simulink model "CubeX_LQR_2D_READ"  (R2016b)
settings: Solver=VariableStepAuto  StartTime=0.0  StopTime=inf  RelTol=1e-3
settings Model: Creator=Wall  LastModifiedBy=Wall

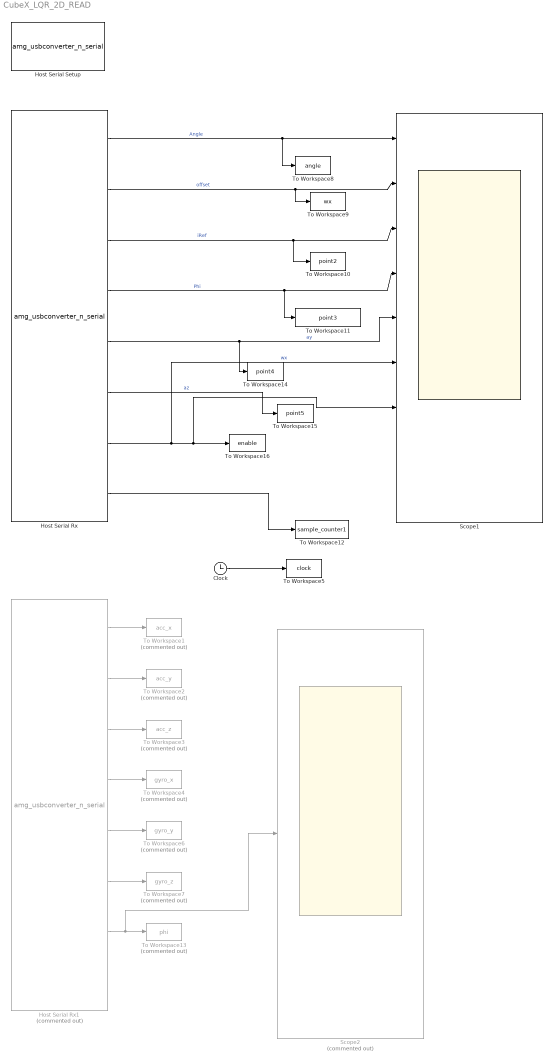
== system CubeX_LQR_2D_READ ==
  Clock : Clock
  Host Serial Rx : S-Function  Priority=1  FunctionName=amg_usbconverter_n_serial  Parameters=configuration,port,transfer,baudrate,stopbit,inputtype,outputtype,binheaderarray,binterminatorarray,asciiheader,asciiterminator,bindatalength,packetmode,timeout,sampletime,initialvalues,blockid  SFunctionDeploymentMode=off  EnableBusSupport=off  mask(amg_usbconverter_n_serial){configuration=Rx, port=COM3, baudrate=115200, databits=8, parity=None, stopbit=1, flowcontrol=None, advanceoptions=off, rxbuffersize=2048, txbuffersize=2048, transfer=Blocking, enableinitial=off, initialvalues=[], timeout=5, packetmode=Binary, binheader='0E 0E', binterminator='0A 0A', porttype_double=8, porttype_single=0, porttype_int8=0, porttype_uint8=0, porttype_int16=0, porttype_uint16=0, porttype_int32=0, porttype_uint32=0, asciiformat='%d,%f', rx_asciiterminator=LF (0x0A - "\n"), tx_asciiterminator=LF (0x0A - "\n"), inputtype=[0], outputtype=[8  0 0 0 0 0 0 0 0], binheaderarray=[2 14  14], binterminatorarray=[2 10  10], bindatalength=64, asciiheader=['%d,%f' uint8(10)], asciiterminator=[1 10], sampletime=0.002, sampletimestr=, blockid=HostSerialRx}
      mask prompts: baudrate "Baud rate (bps)"; databits "Data bits"; stopbit "Stop bit"; flowcontrol "Hardware flow control"; advanceoptions "Advance options"; rxbuffersize "Rx buffer size (bytes)"; txbuffersize "Tx buffer size (bytes)"; enableinitial "Enable initial value  (Closed loop HIL test)"; initialvalues "Initial values"; timeout "Wait time-out (Seconds)"; packetmode "Packet mode"; binheader "Binary header (example: '7E 7E')"; binterminator "Binary terminator (example: '03 03')"; porttype_double "Number of data port, type DOUBLE"; porttype_single "Number of data port, type SINGLE"; porttype_int8 "Number of data port, type INT8"; porttype_uint8 "Number of data port, type UINT8"; porttype_int16 "Number of data port, type INT16"; porttype_uint16 "Number of data port, type UINT16"; porttype_int32 "Number of data port, type INT32"; porttype_uint32 "Number of data port, type UINT32"; asciiformat "Ascii format"; rx_asciiterminator "End of packet"; tx_asciiterminator "End of packet"; inputtype "Input data type"; outputtype "Output data type"; binheaderarray "Binary header"; binterminatorarray "Binary terminator"; bindatalength "Binary data length"; asciiheader "Ascii header (printf format)"; asciiterminator "Ascii terminator"; sampletime "Sample time (sec)"; sampletimestr "Compiled sample time (sec) in string"
      mask help:
      | Enable initial value (Closed loop HIL test):
      |  - Checked: The block will return a initial value (constant) at first time step.
      |  - Unchecked: Normal operation, the block waiting for matched packet data before return value.
      mask init:
      | amg_usbconverter_n_serial_callback('init');
      mask Help: web(fullfile(waijungdocroot,'amg_usbconverter_n_uart.htm'), '-browser')
      mask TypeOptions configuration: Setup | Tx | Rx
      mask Callback configuration: amg_usbconverter_n_serial_callback('configuration');
      mask TypeOptions port: COM3
      mask Callback port: amg_usbconverter_n_serial_callback('port');
      mask Callback baudrate: amg_usbconverter_n_serial_callback('baudrate');
      mask TypeOptions databits: 8
      mask TypeOptions parity: None
      mask TypeOptions stopbit: 1 | 1.5 | 2
      mask TypeOptions flowcontrol: None | RTS | CTS | RTS/CTS
      mask Callback flowcontrol: amg_usbconverter_n_serial_callback('flowcontrol');
      mask Callback advanceoptions: amg_usbconverter_n_serial_callback('advanceoptions');
      mask TypeOptions rxbuffersize: 16 | 32 | 64 | 128 | 256 | 512 | 1024 | 2048
      mask TypeOptions txbuffersize: 16 | 32 | 64 | 128 | 256 | 512 | 1024 | 2048
      mask TypeOptions transfer: Blocking | Non-Blocking
      mask Callback transfer: amg_usbconverter_n_serial_callback('transfer');
      mask Callback enableinitial: amg_usbconverter_n_serial_callback('enableinitial');
      mask Callback initialvalues: amg_usbconverter_n_serial_callback('initialvalues');
      mask TypeOptions packetmode: Ascii | Binary
      mask Callback packetmode: amg_usbconverter_n_serial_callback('packetmode');
      mask Callback binheader: amg_usbconverter_n_serial_callback('binheader');
      mask Callback binterminator: amg_usbconverter_n_serial_callback('binterminator');
      mask Callback porttype_double: amg_usbconverter_n_serial_callback('porttype');
      mask Callback porttype_single: amg_usbconverter_n_serial_callback('porttype');
      mask Callback porttype_int8: amg_usbconverter_n_serial_callback('porttype');
      mask Callback porttype_uint8: amg_usbconverter_n_serial_callback('porttype');
      mask Callback porttype_int16: amg_usbconverter_n_serial_callback('porttype');
      mask Callback porttype_uint16: amg_usbconverter_n_serial_callback('porttype');
      mask Callback porttype_int32: amg_usbconverter_n_serial_callback('porttype');
      mask Callback porttype_uint32: amg_usbconverter_n_serial_callback('porttype');
      mask Callback asciiformat: amg_usbconverter_n_serial_callback('asciiformat');
      mask TypeOptions rx_asciiterminator: CR (0x0D - "\r") | LF (0x0A - "\n") | CRLF (0x0D 0x0A - "\r\n")
      mask Callback rx_asciiterminator: amg_usbconverter_n_serial_callback('rx_asciiterminator');
      mask TypeOptions tx_asciiterminator: CR (0x0D - "\r") | LF (0x0A - "\n") | CRLF (0x0D 0x0A - "\r\n") | None
      mask Callback tx_asciiterminator: amg_usbconverter_n_serial_callback('tx_asciiterminator');
      mask Callback sampletime: amg_usbconverter_n_serial_callback('sampletime');
      mask Callback sampletimestr: amg_usbconverter_n_serial_callback('sampletimestr');
      mask Callback blockid: amg_usbconverter_n_serial_callback('blockid');
      mask Display: text(0.05, 0.5, 'Port: COM3\nPacket: Binary\nTransfer: Blocking\nTs (sec): 0.002','ver','middle','hor','left');port_label('output', 1,'double');port_label('output', 2,'double');port_label('output', 3,'double');port_label('output', 4,'double');port_label('output', 5,'double');port_label('output', 6,'double');port_label('output', 7,'double');port_label('output', 8,'double');
  Host Serial Rx1 : S-Function  Priority=1  Commented=on  FunctionName=amg_usbconverter_n_serial  Parameters=configuration,port,transfer,baudrate,stopbit,inputtype,outputtype,binheaderarray,binterminatorarray,asciiheader,asciiterminator,bindatalength,packetmode,timeout,sampletime,initialvalues,blockid  SFunctionDeploymentMode=off  EnableBusSupport=off  mask(amg_usbconverter_n_serial){configuration=Rx, port=COM3, baudrate=115200, databits=8, parity=None, stopbit=1, flowcontrol=None, advanceoptions=off, rxbuffersize=2048, txbuffersize=2048, transfer=Blocking, enableinitial=off, initialvalues=[], timeout=5, packetmode=Binary, binheader='0E 0E', binterminator='0A 0A', porttype_double=8, porttype_single=0, porttype_int8=0, porttype_uint8=0, porttype_int16=0, porttype_uint16=0, porttype_int32=0, porttype_uint32=0, asciiformat='%d,%f', rx_asciiterminator=LF (0x0A - "\n"), tx_asciiterminator=LF (0x0A - "\n"), inputtype=[0], outputtype=[8  0 0 0 0 0 0 0 0], binheaderarray=[2 14  14], binterminatorarray=[2 10  10], bindatalength=64, asciiheader=['%d,%f' uint8(10)], asciiterminator=[1 10], sampletime=0.002, sampletimestr=, blockid=HostSerialRx1}
      mask prompts: baudrate "Baud rate (bps)"; databits "Data bits"; stopbit "Stop bit"; flowcontrol "Hardware flow control"; advanceoptions "Advance options"; rxbuffersize "Rx buffer size (bytes)"; txbuffersize "Tx buffer size (bytes)"; enableinitial "Enable initial value  (Closed loop HIL test)"; initialvalues "Initial values"; timeout "Wait time-out (Seconds)"; packetmode "Packet mode"; binheader "Binary header (example: '7E 7E')"; binterminator "Binary terminator (example: '03 03')"; porttype_double "Number of data port, type DOUBLE"; porttype_single "Number of data port, type SINGLE"; porttype_int8 "Number of data port, type INT8"; porttype_uint8 "Number of data port, type UINT8"; porttype_int16 "Number of data port, type INT16"; porttype_uint16 "Number of data port, type UINT16"; porttype_int32 "Number of data port, type INT32"; porttype_uint32 "Number of data port, type UINT32"; asciiformat "Ascii format"; rx_asciiterminator "End of packet"; tx_asciiterminator "End of packet"; inputtype "Input data type"; outputtype "Output data type"; binheaderarray "Binary header"; binterminatorarray "Binary terminator"; bindatalength "Binary data length"; asciiheader "Ascii header (printf format)"; asciiterminator "Ascii terminator"; sampletime "Sample time (sec)"; sampletimestr "Compiled sample time (sec) in string"
      mask help:
      | Enable initial value (Closed loop HIL test):
      |  - Checked: The block will return a initial value (constant) at first time step.
      |  - Unchecked: Normal operation, the block waiting for matched packet data before return value.
      mask init:
      | amg_usbconverter_n_serial_callback('init');
      mask Help: web(fullfile(waijungdocroot,'amg_usbconverter_n_uart.htm'), '-browser')
      mask TypeOptions configuration: Setup | Tx | Rx
      mask Callback configuration: amg_usbconverter_n_serial_callback('configuration');
      mask TypeOptions port: COM3
      mask Callback port: amg_usbconverter_n_serial_callback('port');
      mask Callback baudrate: amg_usbconverter_n_serial_callback('baudrate');
      mask TypeOptions databits: 8
      mask TypeOptions parity: None
      mask TypeOptions stopbit: 1 | 1.5 | 2
      mask TypeOptions flowcontrol: None | RTS | CTS | RTS/CTS
      mask Callback flowcontrol: amg_usbconverter_n_serial_callback('flowcontrol');
      mask Callback advanceoptions: amg_usbconverter_n_serial_callback('advanceoptions');
      mask TypeOptions rxbuffersize: 16 | 32 | 64 | 128 | 256 | 512 | 1024 | 2048
      mask TypeOptions txbuffersize: 16 | 32 | 64 | 128 | 256 | 512 | 1024 | 2048
      mask TypeOptions transfer: Blocking | Non-Blocking
      mask Callback transfer: amg_usbconverter_n_serial_callback('transfer');
      mask Callback enableinitial: amg_usbconverter_n_serial_callback('enableinitial');
      mask Callback initialvalues: amg_usbconverter_n_serial_callback('initialvalues');
      mask TypeOptions packetmode: Ascii | Binary
      mask Callback packetmode: amg_usbconverter_n_serial_callback('packetmode');
      mask Callback binheader: amg_usbconverter_n_serial_callback('binheader');
      mask Callback binterminator: amg_usbconverter_n_serial_callback('binterminator');
      mask Callback porttype_double: amg_usbconverter_n_serial_callback('porttype');
      mask Callback porttype_single: amg_usbconverter_n_serial_callback('porttype');
      mask Callback porttype_int8: amg_usbconverter_n_serial_callback('porttype');
      mask Callback porttype_uint8: amg_usbconverter_n_serial_callback('porttype');
      mask Callback porttype_int16: amg_usbconverter_n_serial_callback('porttype');
      mask Callback porttype_uint16: amg_usbconverter_n_serial_callback('porttype');
      mask Callback porttype_int32: amg_usbconverter_n_serial_callback('porttype');
      mask Callback porttype_uint32: amg_usbconverter_n_serial_callback('porttype');
      mask Callback asciiformat: amg_usbconverter_n_serial_callback('asciiformat');
      mask TypeOptions rx_asciiterminator: CR (0x0D - "\r") | LF (0x0A - "\n") | CRLF (0x0D 0x0A - "\r\n")
      mask Callback rx_asciiterminator: amg_usbconverter_n_serial_callback('rx_asciiterminator');
      mask TypeOptions tx_asciiterminator: CR (0x0D - "\r") | LF (0x0A - "\n") | CRLF (0x0D 0x0A - "\r\n") | None
      mask Callback tx_asciiterminator: amg_usbconverter_n_serial_callback('tx_asciiterminator');
      mask Callback sampletime: amg_usbconverter_n_serial_callback('sampletime');
      mask Callback sampletimestr: amg_usbconverter_n_serial_callback('sampletimestr');
      mask Callback blockid: amg_usbconverter_n_serial_callback('blockid');
      mask Display: text(0.05, 0.5, 'Port: COM3\nPacket: Binary\nTransfer: Blocking\nTs (sec): -1','ver','middle','hor','left');port_label('output', 1,'double');port_label('output', 2,'double');port_label('output', 3,'double');port_label('output', 4,'double');port_label('output', 5,'double');port_label('output', 6,'double');port_label('output', 7,'double');port_label('output', 8,'double');
  Host Serial Setup : S-Function  Priority=1  FunctionName=amg_usbconverter_n_serial  Parameters=configuration,port,transfer,baudrate,stopbit,inputtype,outputtype,binheaderarray,binterminatorarray,asciiheader,asciiterminator,bindatalength,packetmode,timeout,sampletime,sampletimestr,blockid  SFunctionDeploymentMode=off  EnableBusSupport=off  mask(amg_usbconverter_n_serial){configuration=Setup, port=COM3, baudrate=115200, databits=8, parity=None, stopbit=1, flowcontrol=None, advanceoptions=on, rxbuffersize=2048, txbuffersize=2048, transfer=Blocking, timeout=5, packetmode=Binary, binheader='7E 7E', binterminator='03 03', porttype_double=1, porttype_single=0, porttype_int8=1, porttype_uint8=0, porttype_int16=0, porttype_uint16=0, porttype_int32=0, porttype_uint32=0, asciiformat='%d,%f', rx_asciiterminator=CRLF (0x0D 0x0A - "\r\n"), tx_asciiterminator=CR (0x0D - "\r"), inputtype=[0], outputtype=[0], binheaderarray=[2 126  126], binterminatorarray=[2 3  3], bindatalength=0, asciiheader='', asciiterminator=[0], sampletime=inf, sampletimestr=, blockid=HostSerialSetup}
      mask prompts: baudrate "Baud rate (bps)"; databits "Data bits"; stopbit "Stop bit"; flowcontrol "Hardware flow control"; advanceoptions "Advance options"; rxbuffersize "Rx buffer size (bytes)"; txbuffersize "Tx buffer size (bytes)"; timeout "Wait time-out (Seconds)"; packetmode "Packet mode"; binheader "Binary header (example: '7E 7E')"; binterminator "Binary terminator (example: '03 03')"; porttype_double "Number of data port, type DOUBLE"; porttype_single "Number of data port, type SINGLE"; porttype_int8 "Number of data port, type INT8"; porttype_uint8 "Number of data port, type UINT8"; porttype_int16 "Number of data port, type INT16"; porttype_uint16 "Number of data port, type UINT16"; porttype_int32 "Number of data port, type INT32"; porttype_uint32 "Number of data port, type UINT32"; asciiformat "Ascii format"; rx_asciiterminator "End of packet"; tx_asciiterminator "End of packet"; inputtype "Input data type"; outputtype "Output data type"; binheaderarray "Binary header"; binterminatorarray "Binary terminator"; bindatalength "Binary data length"; asciiheader "Ascii header (printf format)"; asciiterminator "Ascii terminator"; sampletime "Sample time (sec)"; sampletimestr "Compiled sample time (sec) in string"
      mask init:
      | amg_usbconverter_n_serial_callback('init');
      mask Help: web(fullfile(waijungdocroot,'amg_usbconverter_n_uart.htm'), '-browser')
      mask TypeOptions configuration: Setup | Tx | Rx
      mask Callback configuration: amg_usbconverter_n_serial_callback('configuration');
      mask TypeOptions port: COM3
      mask Callback port: amg_usbconverter_n_serial_callback('port');
      mask Callback baudrate: amg_usbconverter_n_serial_callback('baudrate');
      mask TypeOptions databits: 8
      mask TypeOptions parity: None
      mask TypeOptions stopbit: 1 | 1.5 | 2
      mask TypeOptions flowcontrol: None | RTS | CTS | RTS/CTS
      mask Callback flowcontrol: amg_usbconverter_n_serial_callback('flowcontrol');
      mask Callback advanceoptions: amg_usbconverter_n_serial_callback('advanceoptions');
      mask TypeOptions rxbuffersize: 16 | 32 | 64 | 128 | 256 | 512 | 1024 | 2048
      mask TypeOptions txbuffersize: 16 | 32 | 64 | 128 | 256 | 512 | 1024 | 2048
      mask TypeOptions transfer: Blocking | Non-Blocking
      mask Callback transfer: amg_usbconverter_n_serial_callback('transfer');
      mask TypeOptions packetmode: Ascii | Binary
      mask Callback packetmode: amg_usbconverter_n_serial_callback('packetmode');
      mask Callback binheader: amg_usbconverter_n_serial_callback('binheader');
      mask Callback binterminator: amg_usbconverter_n_serial_callback('binterminator');
      mask Callback porttype_double: amg_usbconverter_n_serial_callback('porttype');
      mask Callback porttype_single: amg_usbconverter_n_serial_callback('porttype');
      mask Callback porttype_int8: amg_usbconverter_n_serial_callback('porttype');
      mask Callback porttype_uint8: amg_usbconverter_n_serial_callback('porttype');
      mask Callback porttype_int16: amg_usbconverter_n_serial_callback('porttype');
      mask Callback porttype_uint16: amg_usbconverter_n_serial_callback('porttype');
      mask Callback porttype_int32: amg_usbconverter_n_serial_callback('porttype');
      mask Callback porttype_uint32: amg_usbconverter_n_serial_callback('porttype');
      mask Callback asciiformat: amg_usbconverter_n_serial_callback('asciiformat');
      mask TypeOptions rx_asciiterminator: CR (0x0D - "\r") | LF (0x0A - "\n") | CRLF (0x0D 0x0A - "\r\n")
      mask Callback rx_asciiterminator: amg_usbconverter_n_serial_callback('rx_asciiterminator');
      mask TypeOptions tx_asciiterminator: CR (0x0D - "\r") | LF (0x0A - "\n") | CRLF (0x0D 0x0A - "\r\n") | None
      mask Callback tx_asciiterminator: amg_usbconverter_n_serial_callback('tx_asciiterminator');
      mask Callback sampletime: amg_usbconverter_n_serial_callback('sampletime');
      mask Callback sampletimestr: amg_usbconverter_n_serial_callback('sampletimestr');
      mask Callback blockid: amg_usbconverter_n_serial_callback('blockid');
      mask Display: text(0.5, 0.5, 'Port: COM3\nBaud (Bps): 115200\nFrame: 8-None-1','ver','middle','hor','center');
  Scope1 : Scope  NumInputPorts=9
  Scope2 : Scope  Commented=on
  To Workspace1 : ToWorkspace  Commented=on  VariableName=acc_x  SaveFormat=Timeseries  SampleTime=-1
  To Workspace10 : ToWorkspace  VariableName=point2  SaveFormat=Timeseries  SampleTime=-1
  To Workspace11 : ToWorkspace  VariableName=point3  SaveFormat=Timeseries  SampleTime=-1
  To Workspace12 : ToWorkspace  VariableName=sample_counter1  SaveFormat=Timeseries  SampleTime=-1
  To Workspace13 : ToWorkspace  Commented=on  VariableName=phi  SaveFormat=Timeseries  SampleTime=-1
  To Workspace14 : ToWorkspace  VariableName=point4  SaveFormat=Timeseries  SampleTime=-1
  To Workspace15 : ToWorkspace  VariableName=point5  SaveFormat=Timeseries  SampleTime=-1
  To Workspace16 : ToWorkspace  VariableName=enable  SaveFormat=Timeseries  SampleTime=-1
  To Workspace2 : ToWorkspace  Commented=on  VariableName=acc_y  SaveFormat=Timeseries  SampleTime=-1
  To Workspace3 : ToWorkspace  Commented=on  VariableName=acc_z  SaveFormat=Timeseries  SampleTime=-1
  To Workspace4 : ToWorkspace  Commented=on  VariableName=gyro_x  SaveFormat=Timeseries  SampleTime=-1
  To Workspace5 : ToWorkspace  VariableName=clock  SaveFormat=Timeseries  SampleTime=-1
  To Workspace6 : ToWorkspace  Commented=on  VariableName=gyro_y  SaveFormat=Timeseries  SampleTime=-1
  To Workspace7 : ToWorkspace  Commented=on  VariableName=gyro_z  SaveFormat=Timeseries  SampleTime=-1
  To Workspace8 : ToWorkspace  VariableName=angle  SaveFormat=Timeseries  SampleTime=-1
  To Workspace9 : ToWorkspace  VariableName=wx  SaveFormat=Timeseries  SampleTime=-1
  wires:
  Clock/1 -> To Workspace5/1
  Host Serial Rx/2 -> To Workspace9/1, Scope1/2  "offset"
  Host Serial Rx/3 -> To Workspace10/1, Scope1/3  "iRef"
  Host Serial Rx/4 -> To Workspace11/1, Scope1/4  "Phi"
  Host Serial Rx/8 -> To Workspace12/1
  Host Serial Rx/1 -> To Workspace8/1, Scope1/1  "Angle"
  Host Serial Rx/5 -> To Workspace14/1, Scope1/5  "ay"
  Host Serial Rx/6 -> To Workspace15/1  "az"
  Host Serial Rx1/1 -> To Workspace1/1
  Host Serial Rx1/2 -> To Workspace2/1
  Host Serial Rx1/3 -> To Workspace3/1
  Host Serial Rx1/4 -> To Workspace4/1
  Host Serial Rx1/5 -> To Workspace6/1
  Host Serial Rx1/6 -> To Workspace7/1
  Host Serial Rx1/7 -> Scope2/1, To Workspace13/1
  Host Serial Rx/7 -> Scope1/6, Scope1/7, To Workspace16/1  "wx"
